simulink model "Flex_Joint"  (R2024b)
settings: Solver=VariableStepAuto  StartTime=0.0  StopTime=60  FixedStep=0.1  RelTol=1e-3  EnableMultiTasking=on
undefined symbols (not defined in the file): Kej4, Kej4b, pert
libraries: simulink x1
settings Model: Creator=AP  LastModifiedBy=dario
settings SolverCC: AlgebraicLoopSolver=TrustRegion
settings DataIOCC: LimitDataPoints=on  SaveFormat=StructureWithTime  SignalLoggingSaveFormat=ModelDataLogs  SaveState=on  ReturnWorkspaceOutputs=off
settings OptimizationCC: ExpressionDepthLimit=2147483647  InitFltsAndDblsToZero=on  LifeSpan=inf
settings DebuggingCC: SaveWithParameterizedLinksMsg=none  UnderspecifiedInitializationDetection=Classic  MergeDetectMultiDrivingBlocksExec=none  FcnCallInpInsideContextMsg=warning  UnconnectedInputMsg=warning  UnconnectedOutputMsg=warning  UnconnectedLineMsg=warning  StateNameClashWarn=warning  SFUnexpectedBacktrackingDiag=warning  SFNoUnconditionalDefaultTransitionDiag=warning  SFExecutionAtInitializationDiag=none  ArithmeticOperatorsInVariantConditions=warning
settings HardwareCC: ProdBitPerPointer=32  ProdBitPerSizeT=32  ProdBitPerPtrDiffT=32  ProdLargestAtomicFloat=None  ProdIntDivRoundTo=Undefined  ProdEndianess=Unspecified  ProdWordSize=32  ProdHWDeviceType=32-bit Generic
settings ModelReferenceCC: EnableRefExpFcnMdlSchedulingChecks=on  PropagateSignalLabelsOutOfModel=off
settings SFSimCC: SimParseCustomCode=off
settings RTWCC: GPUComputeCapability=3.5
settings CodeAppCC: StateflowObjectComments=on
settings GRTTargetCC: TargetFcnLib=ansi_tfl_tmw.mat  TargetLangStandard=C89/C90 (ANSI)  CombineOutputUpdateFcns=off  GRTInterface=on
settings ConfigComp: CovMetricSettings=dw  CovSaveCumulativeToWorkspaceVar=on  CovSaveSingleToWorkspaceVar=on

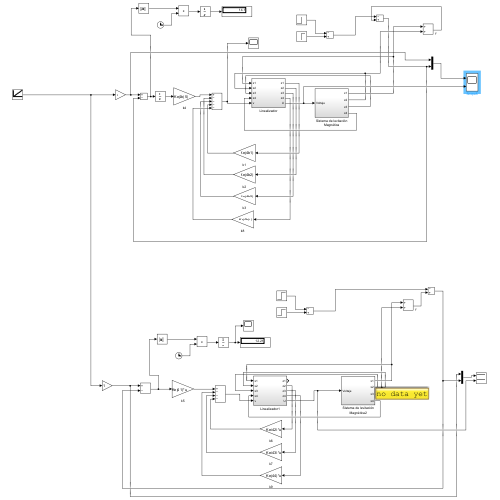
[thumbnail: Simulink's stored preview of the top-level diagram]
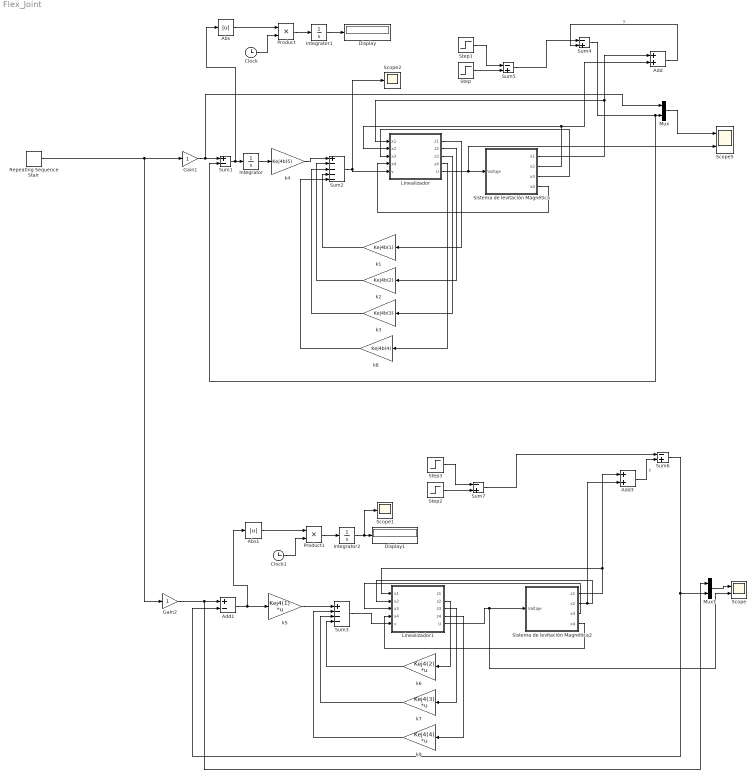
== system Flex_Joint ==
  Abs : Abs  SaturateOnIntegerOverflow=off
  Abs1 : Abs  SaturateOnIntegerOverflow=off
  Add : Sum
  Add1 : Sum  Inputs=+-
  Add3 : Sum
  Clock : Clock
  Clock1 : Clock
  Display : Display
  Display1 : Display
  Gain1 : Gain
  Gain2 : Gain
  Integrator : Integrator
  Integrator1 : Integrator
  Integrator2 : Integrator
  Linealizador : Subsystem
  Linealizador1 : Subsystem
  Mux : Mux  Inputs=2
  Mux1 : Mux  Inputs=2
  Product : Product
  Product1 : Product
  Repeating Sequence Stair : simulink/Sources/Repeating Sequence Stair  OutValues=[0 0.02 0.04 0.06 0.08 0.1 0.12 0.14 0.16 0.18 0.2].'*1  tsamp=4  OutMin=[]  OutMax=[]  OutDataTypeStr=float('double')  OutputDataTypeScalingMode=Specify via dialog  OutDataType=float('double')  ConRadixGroup=Best Precision: Vector-wise  OutScaling=2^-12
  Scope : Scope  NumInputPorts=2
  Scope1 : Scope
  Scope2 : Scope
  Scope5 : Scope  NumInputPorts=2
  Sistema de levitación Magnética : Subsystem
  Sistema de levitación Magnética2 : Subsystem
  Step : Step  Time=5  After=pert  SampleTime=0
  Step1 : Step  Time=5.1  After=pert  SampleTime=0
  Step2 : Step  Time=5  After=pert  SampleTime=0
  Step3 : Step  Time=5.1  After=pert  SampleTime=0
  Sum1 : Sum  Inputs=+-
  Sum2 : Sum  Inputs=+----
  Sum3 : Sum  Inputs=+---
  Sum{4..7} (4 alike) : Sum  Inputs=-+
  k1 : Gain  Gain=Kej4b(1)
  k2 : Gain  Gain=Kej4b(2)
  k3 : Gain  Gain=Kej4b(3)
  k4 : Gain  Gain=Kej4b(5)
  k5 : Gain  Gain=Kej4(1)  Multiplication=Matrix(K*u)
  k6 : Gain  Gain=Kej4(2)  Multiplication=Matrix(K*u)
  k7 : Gain  Gain=Kej4(3)  Multiplication=Matrix(K*u)
  k8 : Gain  Gain=Kej4b(4)
  k9 : Gain  Gain=Kej4(4)  Multiplication=Matrix(K*u)
  wires:
  Sum5/1 -> Sum4/1
  Step/1 -> Sum5/2
  Step1/1 -> Sum5/1
  Gain1/1 -> Sum1/1, Mux/1
  Linealizador/5(U) -> Scope5/2, Sistema de levitación Magnética/1(Voltaje)
  Sistema de levitación Magnética/2(x2) -> Add/2, Linealizador/2(x2)
  Sistema de levitación Magnética/3(x3) -> Linealizador/3(x3)
  Linealizador/2(z2) -> k2/1
  Linealizador/3(z3) -> k3/1
  Sum2/1 -> Linealizador/5(v), Scope2/1
  k2/1 -> Sum2/2
  k3/1 -> Sum2/3
  k4/1 -> Sum2/1
  Linealizador/1(z1) -> k1/1
  k1/1 -> Sum2/4
  Integrator/1 -> k4/1
  Sum1/1 -> Abs/1, Integrator/1
  Sistema de levitación Magnética/4(x4) -> Linealizador/4(x4)
  k8/1 -> Sum2/5
  Linealizador/4(z4) -> k8/1
  Sistema de levitación Magnética/1(x1) -> Add/1, Linealizador/1(x1)
  Mux/1 -> Scope5/1
  Linealizador1/5(U) -> Scope/2, Sistema de levitación Magnética2/1(Voltaje)
  k5/1 -> Sum3/1
  Sum3/1 -> Linealizador1/5(v)
  Sistema de levitación Magnética2/1(x1) -> Add3/1, Linealizador1/1(x1)
  Sistema de levitación Magnética2/2(x2) -> Add3/2, Linealizador1/2(x2)
  Sistema de levitación Magnética2/3(x3) -> Linealizador1/3(x3)
  Sistema de levitación Magnética2/4(x4) -> Linealizador1/4(x4)
  Linealizador1/2(z2) -> k6/1
  Linealizador1/3(z3) -> k7/1
  Linealizador1/4(z4) -> k9/1
  k6/1 -> Sum3/4
  k7/1 -> Sum3/3
  k9/1 -> Sum3/2
  Repeating Sequence Stair/1 -> Gain2/1, Gain1/1
  Sum6/1 -> Mux1/2, Add1/2
  Gain2/1 -> Mux1/1, Add1/1
  Sum4/1 -> Sum1/2, Mux/2
  Add/1 -> Sum4/2  "y"
  Step3/1 -> Sum7/1
  Step2/1 -> Sum7/2
  Sum7/1 -> Sum6/1
  Add3/1 -> Sum6/2  "y"
  Mux1/1 -> Scope/1
  Abs/1 -> Product/1
  Clock/1 -> Product/2
  Product/1 -> Integrator1/1
  Integrator1/1 -> Display/1
  Abs1/1 -> Product1/1
  Product1/1 -> Integrator2/1
  Add1/1 -> Abs1/1, k5/1
  Integrator2/1 -> Scope1/1, Display1/1
  Clock1/1 -> Product1/2

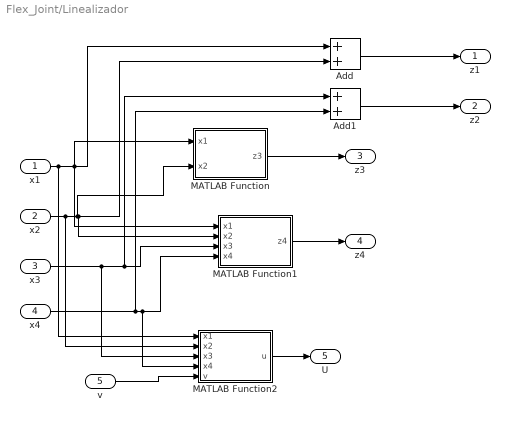
== system Flex_Joint/Linealizador ==
  x1 : Inport
  x2 : Inport  Port=2
  x3 : Inport  Port=3
  x4 : Inport  Port=4
  v : Inport  Port=5
  Add : Sum
  Add1 : Sum
  MATLAB Function : MATLAB Function  TreatAsAtomicUnit=on
  MATLAB Function1 : MATLAB Function  TreatAsAtomicUnit=on
  MATLAB Function2 : MATLAB Function  TreatAsAtomicUnit=on
  z1 : Outport
  z2 : Outport  Port=2
  z3 : Outport  Port=3
  z4 : Outport  Port=4
  U : Outport  Port=5
  wires:
  MATLAB Function2/1(u) -> U/1
  x2/1 -> MATLAB Function2/2(x2), Add/2, MATLAB Function1/2(x2), MATLAB Function/2(x2)
  Add/1 -> z1/1
  x3/1 -> MATLAB Function2/3(x3), Add1/1, MATLAB Function1/3(x3)
  Add1/1 -> z2/1
  x1/1 -> MATLAB Function2/1(x1), Add/1, MATLAB Function1/1(x1), MATLAB Function/1(x1)
  MATLAB Function/1(z3) -> z3/1
  x4/1 -> Add1/2, MATLAB Function2/4(x4), MATLAB Function1/4(x4)
  MATLAB Function1/1(z4) -> z4/1
  v/1 -> MATLAB Function2/5(v)

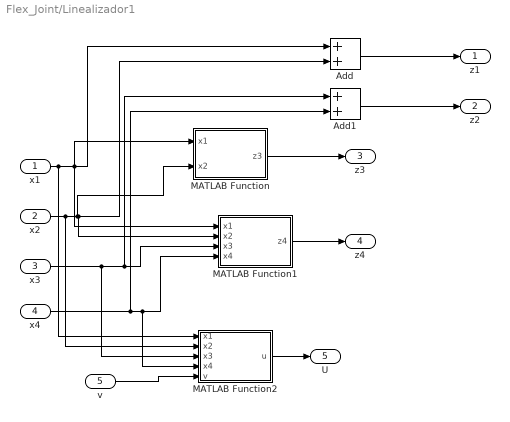
== system Flex_Joint/Linealizador1 ==
  x1 : Inport
  x2 : Inport  Port=2
  x3 : Inport  Port=3
  x4 : Inport  Port=4
  v : Inport  Port=5
  Add : Sum
  Add1 : Sum
  MATLAB Function : MATLAB Function  TreatAsAtomicUnit=on
  MATLAB Function1 : MATLAB Function  TreatAsAtomicUnit=on
  MATLAB Function2 : MATLAB Function  TreatAsAtomicUnit=on
  z1 : Outport
  z2 : Outport  Port=2
  z3 : Outport  Port=3
  z4 : Outport  Port=4
  U : Outport  Port=5
  wires:
  v/1 -> MATLAB Function2/5(v)
  MATLAB Function1/1(z4) -> z4/1
  x4/1 -> Add1/2, MATLAB Function1/4(x4), MATLAB Function2/4(x4)
  MATLAB Function/1(z3) -> z3/1
  x1/1 -> MATLAB Function/1(x1), MATLAB Function1/1(x1), Add/1, MATLAB Function2/1(x1)
  Add1/1 -> z2/1
  x3/1 -> Add1/1, MATLAB Function1/3(x3), MATLAB Function2/3(x3)
  Add/1 -> z1/1
  x2/1 -> MATLAB Function/2(x2), MATLAB Function1/2(x2), Add/2, MATLAB Function2/2(x2)
  MATLAB Function2/1(u) -> U/1

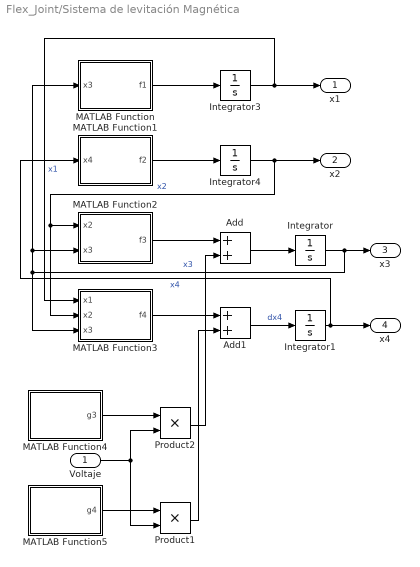
== system Flex_Joint/Sistema de levitación Magnética ==
  Voltaje : Inport
  Add : Sum
  Add1 : Sum
  Integrator{,1,3..4} (4 alike) : Integrator
  MATLAB Function : MATLAB Function  TreatAsAtomicUnit=on
  MATLAB Function1 : MATLAB Function  TreatAsAtomicUnit=on
  MATLAB Function2 : MATLAB Function  TreatAsAtomicUnit=on
  MATLAB Function3 : MATLAB Function  TreatAsAtomicUnit=on
  MATLAB Function4 : MATLAB Function  TreatAsAtomicUnit=on
  MATLAB Function5 : MATLAB Function  TreatAsAtomicUnit=on
  Product1 : Product
  Product2 : Product
  x1 : Outport
  x2 : Outport  Port=2
  x3 : Outport  Port=3
  x4 : Outport  Port=4
  wires:
  MATLAB Function/1(f1) -> Integrator3/1
  MATLAB Function1/1(f2) -> Integrator4/1
  MATLAB Function3/1(f4) -> Add1/1
  MATLAB Function2/1(f3) -> Add/1
  Integrator3/1 -> x1/1, MATLAB Function3/1(x1)  "x1"
  Integrator4/1 -> x2/1, MATLAB Function2/1(x2), MATLAB Function3/2(x2)  "x2"
  Add/1 -> Integrator/1
  Add1/1 -> Integrator1/1  "dx4"
  MATLAB Function4/1(g3) -> Product2/1
  MATLAB Function5/1(g4) -> Product1/1
  Voltaje/1 -> Product2/2, Product1/2
  Product2/1 -> Add/2
  Product1/1 -> Add1/2
  Integrator/1 -> MATLAB Function3/3(x3), MATLAB Function/1(x3), MATLAB Function2/2(x3), x3/1  "x3"
  Integrator1/1 -> MATLAB Function1/1(x4), x4/1  "x4"

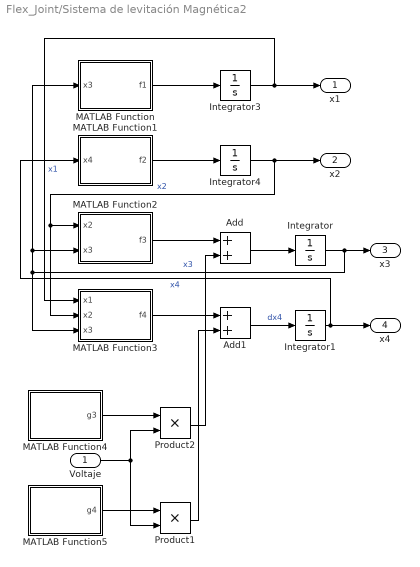
== system Flex_Joint/Sistema de levitación Magnética2 ==
  Voltaje : Inport
  Add : Sum
  Add1 : Sum
  Integrator{,1,3..4} (4 alike) : Integrator
  MATLAB Function : MATLAB Function  TreatAsAtomicUnit=on
  MATLAB Function1 : MATLAB Function  TreatAsAtomicUnit=on
  MATLAB Function2 : MATLAB Function  TreatAsAtomicUnit=on
  MATLAB Function3 : MATLAB Function  TreatAsAtomicUnit=on
  MATLAB Function4 : MATLAB Function  TreatAsAtomicUnit=on
  MATLAB Function5 : MATLAB Function  TreatAsAtomicUnit=on
  Product1 : Product
  Product2 : Product
  x1 : Outport
  x2 : Outport  Port=2
  x3 : Outport  Port=3
  x4 : Outport  Port=4
  wires:
  MATLAB Function/1(f1) -> Integrator3/1
  MATLAB Function1/1(f2) -> Integrator4/1
  MATLAB Function3/1(f4) -> Add1/1
  MATLAB Function2/1(f3) -> Add/1
  Integrator3/1 -> x1/1, MATLAB Function3/1(x1)  "x1"
  Integrator4/1 -> x2/1, MATLAB Function2/1(x2), MATLAB Function3/2(x2)  "x2"
  Add/1 -> Integrator/1
  Add1/1 -> Integrator1/1  "dx4"
  MATLAB Function4/1(g3) -> Product2/1
  MATLAB Function5/1(g4) -> Product1/1
  Voltaje/1 -> Product2/2, Product1/2
  Product2/1 -> Add/2
  Product1/1 -> Add1/2
  Integrator/1 -> MATLAB Function3/3(x3), MATLAB Function/1(x3), MATLAB Function2/2(x3), x3/1  "x3"
  Integrator1/1 -> MATLAB Function1/1(x4), x4/1  "x4"

== matlab function Flex_Joint/Linealizador1/MATLAB Function2 ==
  data: x1 input; u output; x2 input; x3 input; x4 input; v input
function u = fcn(x1,x2,x3,x4,v)

Ks = 1.61;         % Rigidez del resorte [N/m]
Jh = 0.0021;       % Inercia del eje del motor [kg*m^2]
m = 0.403;         % Masa del brazo [kg]
g = -9.81;         % Aceleración de la gravedad [m/s^2]
h = 0.06;          % Altura del centro de masa [m]
Km = 0.00767;      % Constante del motor [N·rad/s]
Kg = 70;           % Relación de engranaje
Jl = 0.0059;       % Inercia de la carga [kg*m^2]
Rm = 2.6;          % Resistencia del motor [Ohm]

u = (Jh*Jl^2*Rm*v - Jh*Ks^2*Rm*x2 - Jl*Ks^2*Rm*x2 + Jl*Kg^2*Km^2*Ks*x3 - (Jh*Rm*g^2*h^2*m^2*sin(2*x1 + 2*x2))/2 + Jh*Ks*Rm*g*h*m*sin(x1 + x2) + Jh*Jl*Rm*g*h*m*x3^2*sin(x1 + x2) + Jh*Jl*Rm*g*h*m*x4^2*sin(x1 + x2) + Jh*Ks*Rm*g*h*m*x2*cos(x1 + x2) + 2*Jh*Jl*Rm*g*h*m*x3*x4*sin(x1 + x2))/(Jl*Kg*Km*Ks);

== matlab function Flex_Joint/Sistema de levitación Magnética/MATLAB Function1 ==
  data: x4 input; f2 output
function f2 = fcn(x4)

f2 = x4;

== matlab function Flex_Joint/Sistema de levitación Magnética2/MATLAB Function ==
  data: x3 input; f1 output
function f1 = fcn(x3)

f1 = x3;

== matlab function Flex_Joint/Sistema de levitación Magnética2/MATLAB Function1 ==
  data: x4 input; f2 output
function f2 = fcn(x4)

f2 = x4;

== matlab function Flex_Joint/Sistema de levitación Magnética2/MATLAB Function2 ==
  data: x2 input; f3 output; x3 input
function f3 = fcn(x2,x3)
Ks = 1.61;         % Rigidez del resorte [N/m]
Jh = 0.0021;       % Inercia del eje del motor [kg*m^2]
g = -9.81;         % Aceleración de la gravedad [m/s^2]
Km = 0.00767;      % Constante del motor [N·rad/s]
Kg = 70;           % Relación de engranaje
Rm = 2.6;          % Resistencia del motor [Ohm]

f3 = ( Ks / Jh )*x2 - ( Km^2 * Kg^2 / (Rm * Jh) )*x3;

== matlab function Flex_Joint/Sistema de levitación Magnética2/MATLAB Function3 ==
  data: x1 input; x2 input; f4 output; x3 input
function f4 = fcn(x1,x2,x3)
Ks = 1.61;         % Rigidez del resorte [N/m]
Jh = 0.0021;       % Inercia del eje del motor [kg*m^2]
m = 0.403;         % Masa del brazo [kg]
g = -9.81;         % Aceleración de la gravedad [m/s^2]
h = 0.06;          % Altura del centro de masa [m]
Km = 0.00767;      % Constante del motor [N·rad/s]
Kg = 70;           % Relación de engranaje
Jl = 0.0059;       % Inercia de la carga [kg*m^2]
Rm = 2.6;          % Resistencia del motor [Ohm]

f4 = -( Ks/Jh + Ks/Jl )*x2 + ( m * g * h / Jl )*sin( x1 + x2 ) + ( Km^2 * Kg^2 / (Rm * Jh) )*x3;

== matlab function Flex_Joint/Sistema de levitación Magnética2/MATLAB Function4 ==
  data: g3 output
function g3 = fcn

Jh = 0.0021;       % Inercia del eje del motor [kg*m^2]
g = -9.81;         % Aceleración de la gravedad [m/s^2]
Km = 0.00767;      % Constante del motor [N·rad/s]
Kg = 70;           % Relación de engranaje
Rm = 2.6;          % Resistencia del motor [Ohm]


g3 = Km * Kg / (Rm * Jh);

== matlab function Flex_Joint/Sistema de levitación Magnética2/MATLAB Function5 ==
  data: g4 output
function g4 = fcn

Jh = 0.0021;       % Inercia del eje del motor [kg*m^2]
g = -9.81;         % Aceleración de la gravedad [m/s^2]
Km = 0.00767;      % Constante del motor [N·rad/s]
Kg = 70;           % Relación de engranaje
Rm = 2.6;          % Resistencia del motor [Ohm]


g4 = -( Km * Kg / (Rm * Jh) );

== matlab function Flex_Joint/Sistema de levitación Magnética/MATLAB Function ==
  data: x3 input; f1 output
function f1 = fcn(x3)

f1 = x3;

== matlab function Flex_Joint/Sistema de levitación Magnética/MATLAB Function2 ==
  data: x2 input; f3 output; x3 input
function f3 = fcn(x2,x3)
Ks = 1.61;         % Rigidez del resorte [N/m]
Jh = 0.0021;       % Inercia del eje del motor [kg*m^2]
g = -9.81;         % Aceleración de la gravedad [m/s^2]
Km = 0.00767;      % Constante del motor [N·rad/s]
Kg = 70;           % Relación de engranaje
Rm = 2.6;          % Resistencia del motor [Ohm]

f3 = ( Ks / Jh )*x2 - ( Km^2 * Kg^2 / (Rm * Jh) )*x3;

== matlab function Flex_Joint/Sistema de levitación Magnética/MATLAB Function3 ==
  data: x1 input; x2 input; f4 output; x3 input
function f4 = fcn(x1,x2,x3)
Ks = 1.61;         % Rigidez del resorte [N/m]
Jh = 0.0021;       % Inercia del eje del motor [kg*m^2]
m = 0.403;         % Masa del brazo [kg]
g = -9.81;         % Aceleración de la gravedad [m/s^2]
h = 0.06;          % Altura del centro de masa [m]
Km = 0.00767;      % Constante del motor [N·rad/s]
Kg = 70;           % Relación de engranaje
Jl = 0.0059;       % Inercia de la carga [kg*m^2]
Rm = 2.6;          % Resistencia del motor [Ohm]

f4 = -( Ks/Jh + Ks/Jl )*x2 + ( m * g * h / Jl )*sin( x1 + x2 ) + ( Km^2 * Kg^2 / (Rm * Jh) )*x3;

== matlab function Flex_Joint/Sistema de levitación Magnética/MATLAB Function4 ==
  data: g3 output
function g3 = fcn

Jh = 0.0021;       % Inercia del eje del motor [kg*m^2]
g = -9.81;         % Aceleración de la gravedad [m/s^2]
Km = 0.00767;      % Constante del motor [N·rad/s]
Kg = 70;           % Relación de engranaje
Rm = 2.6;          % Resistencia del motor [Ohm]


g3 = Km * Kg / (Rm * Jh);

== matlab function Flex_Joint/Sistema de levitación Magnética/MATLAB Function5 ==
  data: g4 output
function g4 = fcn

Jh = 0.0021;       % Inercia del eje del motor [kg*m^2]
g = -9.81;         % Aceleración de la gravedad [m/s^2]
Km = 0.00767;      % Constante del motor [N·rad/s]
Kg = 70;           % Relación de engranaje
Rm = 2.6;          % Resistencia del motor [Ohm]


g4 = -( Km * Kg / (Rm * Jh) );

== matlab function Flex_Joint/Linealizador1/MATLAB Function ==
  data: x1 input; z3 output; x2 input
function z3 = fcn(x1, x2)

Ks = 1.61;         % Rigidez del resorte [N/m]
Jh = 0.0021;       % Inercia del eje del motor [kg*m^2]
m = 0.403;         % Masa del brazo [kg]
g = -9.81;         % Aceleración de la gravedad [m/s^2]
h = 0.06;          % Altura del centro de masa [m]
Jl = 0.0059;       % Inercia de la carga [kg*m^2]

z3 = (Ks*x2)/Jh - x2*(Ks/Jh + Ks/Jl) + (g*h*m*sin(x1 + x2))/Jl;

== matlab function Flex_Joint/Linealizador/MATLAB Function ==
  data: x1 input; z3 output; x2 input
function z3 = fcn(x1, x2)

Ks = 1.61;         % Rigidez del resorte [N/m]
Jh = 0.0021;       % Inercia del eje del motor [kg*m^2]
m = 0.403;         % Masa del brazo [kg]
g = -9.81;         % Aceleración de la gravedad [m/s^2]
h = 0.06;          % Altura del centro de masa [m]
Jl = 0.0059;       % Inercia de la carga [kg*m^2]

z3 = (Ks*x2)/Jh - x2*(Ks/Jh + Ks/Jl) + (g*h*m*sin(x1 + x2))/Jl;

== matlab function Flex_Joint/Linealizador/MATLAB Function1 ==
  data: x1 input; z4 output; x2 input; x3 input; x4 input
function z4 = fcn(x1,x2,x3,x4)
Ks = 1.61;         % Rigidez del resorte [N/m]
m = 0.403;         % Masa del brazo [kg]
g = -9.81;         % Aceleración de la gravedad [m/s^2]
h = 0.06;          % Altura del centro de masa [m]
Jl = 0.0059;       % Inercia de la carga [kg*m^2]

z4 = (g*h*m*x3*cos(x1 + x2))/Jl - x4*(Ks/Jl - (g*h*m*cos(x1 + x2))/Jl);

== matlab function Flex_Joint/Linealizador/MATLAB Function2 ==
  data: x1 input; u output; x2 input; x3 input; x4 input; v input
function u = fcn(x1,x2,x3,x4,v)

Ks = 1.61;         % Rigidez del resorte [N/m]
Jh = 0.0021;       % Inercia del eje del motor [kg*m^2]
m = 0.403;         % Masa del brazo [kg]
g = -9.81;         % Aceleración de la gravedad [m/s^2]
h = 0.06;          % Altura del centro de masa [m]
Km = 0.00767;      % Constante del motor [N·rad/s]
Kg = 70;           % Relación de engranaje
Jl = 0.0059;       % Inercia de la carga [kg*m^2]
Rm = 2.6;          % Resistencia del motor [Ohm]

u = (Jh*Jl^2*Rm*v - Jh*Ks^2*Rm*x2 - Jl*Ks^2*Rm*x2 + Jl*Kg^2*Km^2*Ks*x3 - (Jh*Rm*g^2*h^2*m^2*sin(2*x1 + 2*x2))/2 + Jh*Ks*Rm*g*h*m*sin(x1 + x2) + Jh*Jl*Rm*g*h*m*x3^2*sin(x1 + x2) + Jh*Jl*Rm*g*h*m*x4^2*sin(x1 + x2) + Jh*Ks*Rm*g*h*m*x2*cos(x1 + x2) + 2*Jh*Jl*Rm*g*h*m*x3*x4*sin(x1 + x2))/(Jl*Kg*Km*Ks);

== matlab function Flex_Joint/Linealizador1/MATLAB Function1 ==
  data: x1 input; z4 output; x2 input; x3 input; x4 input
function z4 = fcn(x1,x2,x3,x4)
Ks = 1.61;         % Rigidez del resorte [N/m]
m = 0.403;         % Masa del brazo [kg]
g = -9.81;         % Aceleración de la gravedad [m/s^2]
h = 0.06;          % Altura del centro de masa [m]
Jl = 0.0059;       % Inercia de la carga [kg*m^2]

z4 = (g*h*m*x3*cos(x1 + x2))/Jl - x4*(Ks/Jl - (g*h*m*cos(x1 + x2))/Jl);
